simulink model "LAB2_2_DirectDigitalSignal"  (R2025b)
settings: Solver=FixedStepAuto  StartTime=0.0  StopTime=10  FixedStep=0.0001  RelTol=1e-3
values from neighbouring files (symbols this model uses):
  gamma_o = [gamma(2)-L*gamma(1), (phi22-L*phi12)*L+phi21-L*phi11]    [LAB2_2DirectDigitalSignale.m]
  Ho = [0;1]    [LAB2_2DirectDigitalSignale.m]
  Jo = [0 1; 0 L]    [LAB2_2DirectDigitalSignale.m]
  K = Ke(2:3)    [LAB2_2DirectDigitalSignale.m]
  Ki = Ke(1)    [LAB2_2DirectDigitalSignale.m]
  Nr = Nu + K * Nx    [LAB2_2DirectDigitalSignale.m]
  phi_o = lambda_o_dt    [LAB2_2DirectDigitalSignale.m]
  step_amplitude = 50    [LAB2_2DirectDigitalSignale.m]
  T = input('Select sample time (0.001, 0.01, 0.05) [s]: ')    [LAB2_2DirectDigitalSignale.m]
undefined symbols (not defined in the file or in its folder): Beq, daq, DiscIntNeverNeededParam, drv, gbox, Jeq, mot, pulse2deg, rads2rpm, Req, tau_sf_est
settings Model: Creator=ester  LastModifiedBy=ester

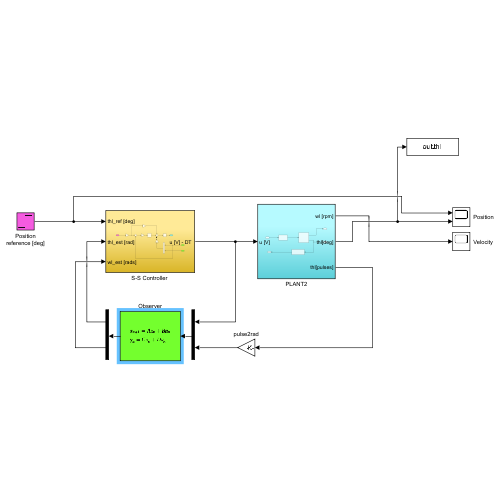
[thumbnail: Simulink's stored preview of the top-level diagram]
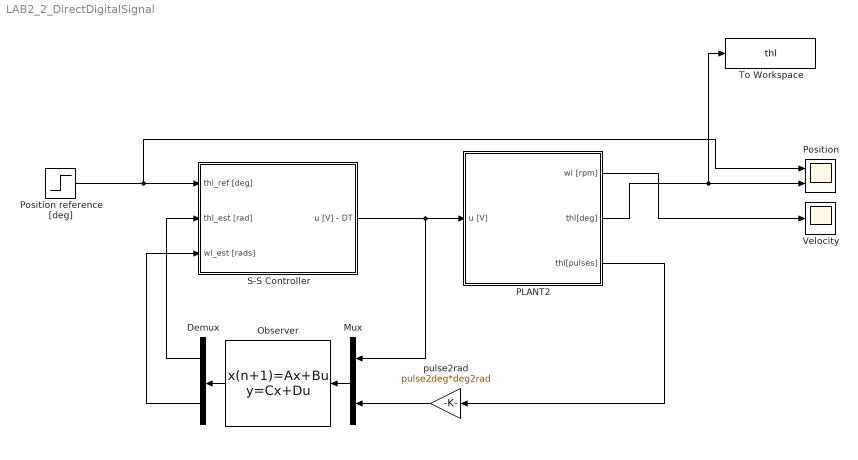
== system LAB2_2_DirectDigitalSignal ==
  Demux : Demux  Outputs=2
  Mux : Mux  Inputs=2
  Observer : DiscreteStateSpace  A=phi_o  B=gamma_o  C=Ho  D=Jo  SampleTime=T
  PLANT2 : Subsystem
  Position : Scope  NumInputPorts=2
      settings: ActiveDisplayYMinimum=-6.5609756966733555  ActiveDisplayYMaximum=59.048781270060218
  Position reference [deg] : Step  After=step_amplitude  SampleTime=T  ZeroCross=off
  "S-S Controller " : Subsystem
  To Workspace : ToWorkspace  VariableName=thl  SampleTime=T
  Velocity : Scope
      settings: ActiveDisplayYMinimum=-1  ActiveDisplayYMaximum=1
  pulse2rad : Gain  Gain=pulse2deg*deg2rad
  wires:
  Position reference [deg]/1 -> "S-S Controller "/1(thl_ref [deg]), Position/1
  Observer/1 -> Demux/1
  Demux/2 -> "S-S Controller "/3(wl_est [rads])
  Demux/1 -> "S-S Controller "/2(thl_est [rad])
  PLANT2/2(thl[deg]) -> To Workspace/1, Position/2
  Mux/1 -> Observer/1
  PLANT2/1(wl [rpm]) -> Velocity/1
  PLANT2/3(thl[pulses]) -> pulse2rad/1
  "S-S Controller "/1("u [V] - DT ") -> PLANT2/1(u [V]), Mux/1
  pulse2rad/1 -> Mux/2

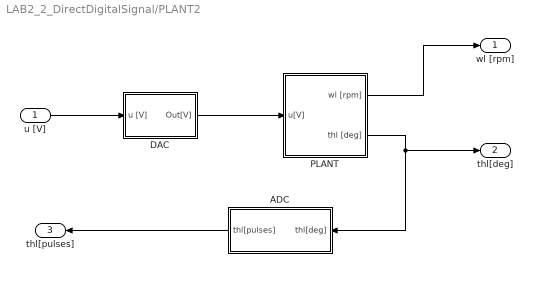
== system LAB2_2_DirectDigitalSignal/PLANT2 ==
  u [V] : Inport
  ADC : Subsystem  TreatAsAtomicUnit=on
  DAC : Subsystem  TreatAsAtomicUnit=on
  PLANT : Subsystem
  wl [rpm] : Outport
  thl[deg] : Outport  Port=2
  thl[pulses] : Outport  Port=3
  wires:
  DAC/1(Out[V]) -> PLANT/1(u[V])
  PLANT/2(thl [deg]) -> thl[deg]/1, ADC/1(thl[deg])
  ADC/1(thl[pulses]) -> thl[pulses]/1
  u [V]/1 -> DAC/1(u [V])
  PLANT/1(wl [rpm]) -> wl [rpm]/1

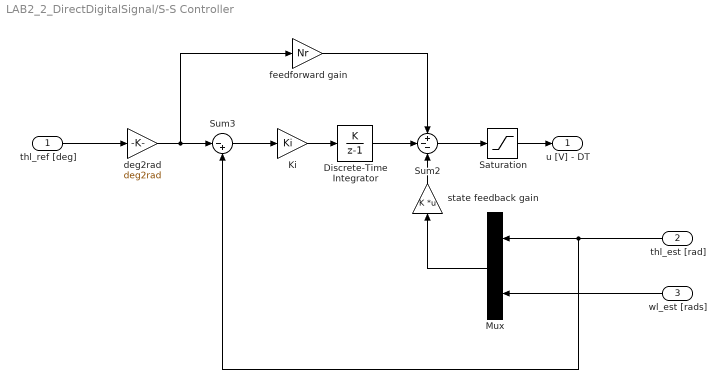
== system LAB2_2_DirectDigitalSignal/S-S Controller  ==
  thl_ref [deg] : Inport
  thl_est [rad] : Inport  Port=2
  wl_est [rads] : Inport  Port=3
  " feedforward gain" : Gain  Gain=Nr
  Discrete-Time Integrator : DiscreteIntegrator  IntegratorMethod=Accumulation: Forward Euler  SampleTime=T  ICPrevOutput=DiscIntNeverNeededParam  ICPrevScaledInput=DiscIntNeverNeededParam
  Ki : Gain  Gain=Ki
  Mux : Mux  Inputs=2
  Saturation : Saturate  UpperLimit=10  LowerLimit=-10  ZeroCross=off
  Sum2 : Sum  Inputs=+--
  Sum3 : Sum  Inputs=|-+
  deg2rad : Gain  Gain=deg2rad
  state feedback gain : Gain  Gain=K  Multiplication=Matrix(K*u)
  "u [V] - DT " : Outport
  wires:
  Mux/1 -> state feedback gain/1
  Ki/1 -> Discrete-Time Integrator/1
  deg2rad/1 -> " feedforward gain"/1, Sum3/1
  Sum2/1 -> Saturation/1
  Saturation/1 -> "u [V] - DT "/1
  thl_est [rad]/1 -> Sum3/2, Mux/1
  Sum3/1 -> Ki/1
  state feedback gain/1 -> Sum2/3
  " feedforward gain"/1 -> Sum2/1
  thl_ref [deg]/1 -> deg2rad/1
  wl_est [rads]/1 -> Mux/2
  Discrete-Time Integrator/1 -> Sum2/2

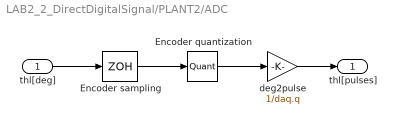
== system LAB2_2_DirectDigitalSignal/PLANT2/ADC ==
  thl[deg] : Inport
  Encoder quantization : Quantizer  QuantizationInterval=daq.q
  Encoder sampling : ZeroOrderHold  SampleTime=daq.dac.Ts
  deg2pulse : Gain  Gain=1/daq.q
  thl[pulses] : Outport
  wires:
  Encoder quantization/1 -> deg2pulse/1
  thl[deg]/1 -> Encoder sampling/1
  Encoder sampling/1 -> Encoder quantization/1
  deg2pulse/1 -> thl[pulses]/1

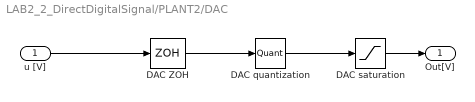
== system LAB2_2_DirectDigitalSignal/PLANT2/DAC ==
  u [V] : Inport
  "DAC ZOH " : ZeroOrderHold  SampleTime=daq.dac.Ts
  DAC quantization : Quantizer  QuantizationInterval=daq.dac.q
  DAC saturation : Saturate  UpperLimit=daq.dac.fs  LowerLimit=-daq.dac.fs
  Out[V] : Outport
  wires:
  DAC quantization/1 -> DAC saturation/1
  u [V]/1 -> "DAC ZOH "/1
  "DAC ZOH "/1 -> DAC quantization/1
  DAC saturation/1 -> Out[V]/1

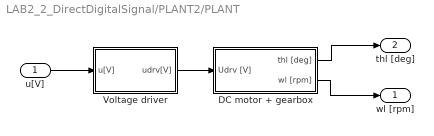
== system LAB2_2_DirectDigitalSignal/PLANT2/PLANT ==
  u[V] : Inport
  DC motor + gearbox : Subsystem
  Voltage driver : Subsystem  TreatAsAtomicUnit=on
  wl [rpm] : Outport
  thl [deg] : Outport  Port=2
  wires:
  Voltage driver/1(udrv[V]) -> DC motor + gearbox/1(Udrv [V])
  u[V]/1 -> Voltage driver/1(u[V])
  DC motor + gearbox/1(thl [deg]) -> thl [deg]/1
  DC motor + gearbox/2(wl [rpm]) -> wl [rpm]/1

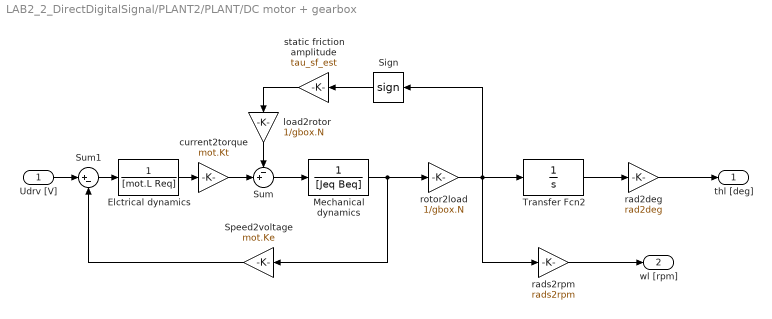
== system LAB2_2_DirectDigitalSignal/PLANT2/PLANT/DC motor + gearbox ==
  Udrv [V] : Inport
  Elctrical dynamics : TransferFcn  Denominator=[mot.L Req]
  Mechanical dynamics : TransferFcn  Denominator=[Jeq Beq]
  Sign : Signum  ZeroCross=off
  Speed2voltage : Gain  Gain=mot.Ke
  Sum : Sum  Inputs=-+|
  Sum1 : Sum  Inputs=|+-
  Transfer Fcn2 : TransferFcn  Denominator=[1 0]
  current2torque : Gain  Gain=mot.Kt
  load2rotor : Gain  Gain=1/gbox.N
  rad2deg : Gain  Gain=rad2deg
  rads2rpm : Gain  Gain=rads2rpm
  rotor2load : Gain  Gain=1/gbox.N
  static friction amplitude : Gain  Gain=tau_sf_est
  thl [deg] : Outport
  wl [rpm] : Outport  Port=2
  wires:
  rotor2load/1 -> Sign/1, rads2rpm/1, Transfer Fcn2/1
  Sign/1 -> static friction amplitude/1
  rads2rpm/1 -> wl [rpm]/1
  Sum/1 -> Mechanical dynamics/1
  Udrv [V]/1 -> Sum1/1
  static friction amplitude/1 -> load2rotor/1
  load2rotor/1 -> Sum/1
  Transfer Fcn2/1 -> rad2deg/1
  current2torque/1 -> Sum/2
  Speed2voltage/1 -> Sum1/2
  Mechanical dynamics/1 -> Speed2voltage/1, rotor2load/1
  Elctrical dynamics/1 -> current2torque/1
  Sum1/1 -> Elctrical dynamics/1
  rad2deg/1 -> thl [deg]/1

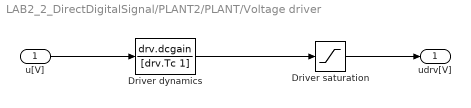
== system LAB2_2_DirectDigitalSignal/PLANT2/PLANT/Voltage driver ==
  u[V] : Inport
  Driver dynamics : TransferFcn  Numerator=drv.dcgain  Denominator=[drv.Tc 1]
  Driver saturation : Saturate  UpperLimit=drv.outmax  LowerLimit=-drv.outmax
  udrv[V] : Outport
  wires:
  Driver dynamics/1 -> Driver saturation/1
  u[V]/1 -> Driver dynamics/1
  Driver saturation/1 -> udrv[V]/1
